simulink model "vertical_dynamics"  (R2025a)
settings: Solver=VariableStepAuto  StartTime=0.0  StopTime=10.0  RelTol=1e-3
InitFcn:
  | vehicleData = read_json(simConfig.vehicleConfigFile);
  | assign_vehicle_params(simConfig.model, vehicleData);
  | set_springDeflection_bus();
model workspace (MAT data in the model file):
  BusSpringDeflection = Simulink.Bus
  BusSpringDeflection.Alignment = -1
  BusSpringDeflection.PreserveElementDimensions = 0
  BusSpringDeflection.Elements_internal(1) = Simulink.BusElement
  BusSpringDeflection.Elements_internal(1).DimensionsMode = 'Fixed'
  BusSpringDeflection.Elements_internal(1).SamplingMode = 'Sample based'
  BusSpringDeflection.Elements_internal(1).SampleTime = -1
  BusSpringDeflection.Elements_internal(1).DocUnits = 'mm'
  BusSpringDeflection.Elements_internal(1).Name = 'springDeflection_FL'
  BusSpringDeflection.Elements_internal(1).DataType_internal = 'double'
  BusSpringDeflection.Elements_internal(1).Complexity = 'real'
  BusSpringDeflection.Elements_internal(1).Dimensions = 1
  BusSpringDeflection.Elements_internal(2) = Simulink.BusElement
  BusSpringDeflection.Elements_internal(2).DimensionsMode = 'Fixed'
  BusSpringDeflection.Elements_internal(2).SamplingMode = 'Sample based'
  BusSpringDeflection.Elements_internal(2).SampleTime = -1
  BusSpringDeflection.Elements_internal(2).DocUnits = 'mm'
  BusSpringDeflection.Elements_internal(2).Name = 'springDeflection_FR'
  BusSpringDeflection.Elements_internal(2).DataType_internal = 'double'
  BusSpringDeflection.Elements_internal(2).Complexity = 'real'
  BusSpringDeflection.Elements_internal(2).Dimensions = 1
  BusSpringDeflection.Elements_internal(3) = Simulink.BusElement
  BusSpringDeflection.Elements_internal(3).DimensionsMode = 'Fixed'
  BusSpringDeflection.Elements_internal(3).SamplingMode = 'Sample based'
  BusSpringDeflection.Elements_internal(3).SampleTime = -1
  BusSpringDeflection.Elements_internal(3).DocUnits = 'mm'
  BusSpringDeflection.Elements_internal(3).Name = 'springDeflection_RL'
  BusSpringDeflection.Elements_internal(3).DataType_internal = 'double'
  BusSpringDeflection.Elements_internal(3).Complexity = 'real'
  BusSpringDeflection.Elements_internal(3).Dimensions = 1
  BusSpringDeflection.Elements_internal(4) = Simulink.BusElement
  BusSpringDeflection.Elements_internal(4).DimensionsMode = 'Fixed'
  BusSpringDeflection.Elements_internal(4).SamplingMode = 'Sample based'
  BusSpringDeflection.Elements_internal(4).SampleTime = -1
  BusSpringDeflection.Elements_internal(4).DocUnits = 'mm'
  BusSpringDeflection.Elements_internal(4).Name = 'springDeflection_RR'
  BusSpringDeflection.Elements_internal(4).DataType_internal = 'double'
  BusSpringDeflection.Elements_internal(4).Complexity = 'real'
  BusSpringDeflection.Elements_internal(4).Dimensions = 1
  BusSpringDeflection.DataScope = 'Auto'
  l = 2975
  lnzv = 1487
  sh = 1587
  sv = 1587
settings Model: Creator=marce  LastModifiedBy=marce

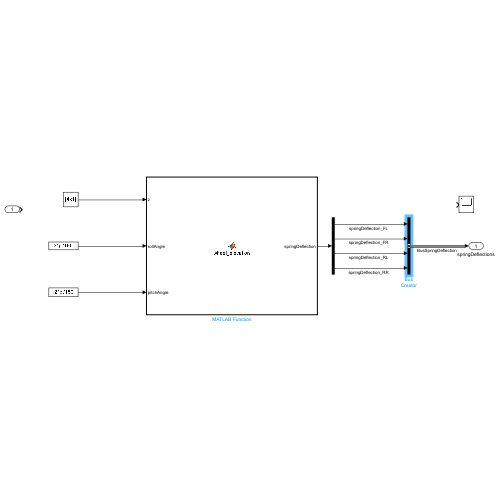
[thumbnail: Simulink's stored preview of the top-level diagram]
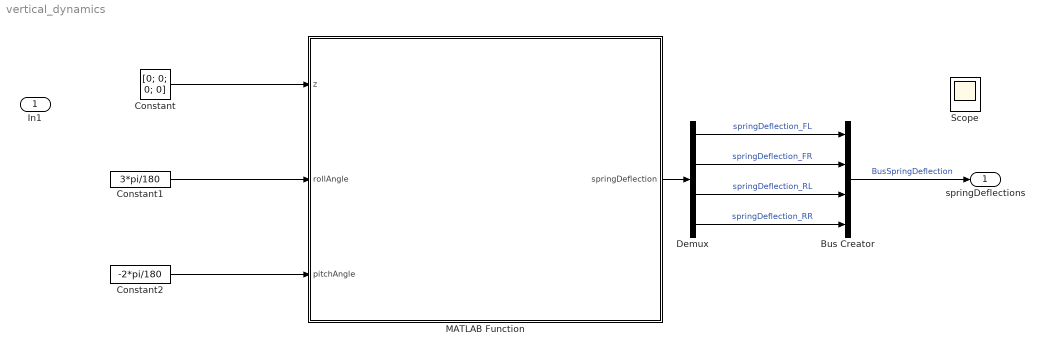
== system vertical_dynamics ==
  In1 : Inport
  Bus Creator : BusCreator  Inputs=4  OutDataTypeStr=Bus: BusObject
  Constant : Constant  Value=[0; 0; 0; 0]
  Constant1 : Constant  Value=3*pi/180
  Constant2 : Constant  Value=-2*pi/180
  Demux : Demux
  MATLAB Function : MATLAB Function  TreatAsAtomicUnit=on
  Scope : Scope
      settings: ActiveDisplayYMinimum=-116.78452853133139  ActiveDisplayYMaximum=116.8194280280339
  springDeflections : Outport
  wires:
  Constant/1 -> MATLAB Function/1(z)
  Constant1/1 -> MATLAB Function/2(rollAngle)
  Constant2/1 -> MATLAB Function/3(pitchAngle)
  MATLAB Function/1(springDeflection) -> Demux/1
  Demux/1 -> Bus Creator/1  "springDeflection_FL"
  Demux/2 -> Bus Creator/2  "springDeflection_FR"
  Demux/3 -> Bus Creator/3  "springDeflection_RL"
  Demux/4 -> Bus Creator/4  "springDeflection_RR"
  Bus Creator/1 -> springDeflections/1  "BusSpringDeflection"

== matlab function vertical_dynamics/MATLAB Function ==
  data: z input; rollAngle input; springDeflection output; pitchAngle input; l parameter double; lnzv parameter double; sh parameter; sv parameter
function springDeflection = wheel_elevation(z, rollAngle, pitchAngle, l, lnzv, sh, sv)

c = 0.5 * (-1).^[1:4]';

trackMultipliers = [sv; sv; sh; sh];
pitchMultipliers = [lnzv; lnzv; (lnzv-l); (lnzv-l)];

springDeflection = z .* ones(4,1) ...
                   + sin(rollAngle) .* (c .* trackMultipliers) ...
                   + sin(pitchAngle) .* pitchMultipliers;
